simulink model "mod4"  (R2017a)
settings: Solver=VariableStepAuto  StartTime=0.0  StopTime=10.0  RelTol=1e-3
libraries: simulink x2
settings Model: Creator=step_oda  LastModifiedBy=step_oda

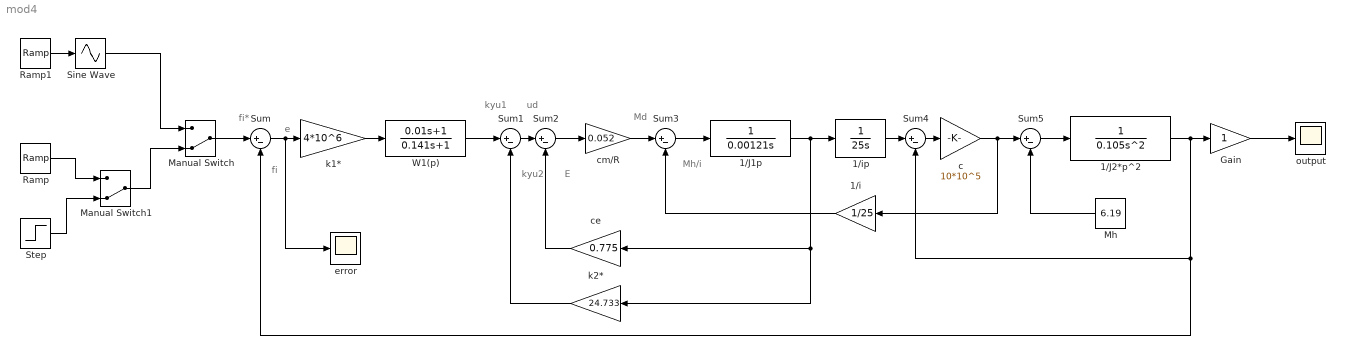
== system mod4 ==
  note: ud
  note: Md
  note: fi
  note: e
  note: fi*
  note: kyu1
  note: kyu2
  note: E
  note: Mh/i
  1/J1p : TransferFcn  Denominator=[0.00121 0]
  1/J2*p^2 : TransferFcn  Denominator=[0.105 0 0]
  1/i : Gain  Gain=1/25
  1/ip : TransferFcn  Denominator=[25 0]
  Gain : Gain
  Manual Switch : ManualSwitch  CurrentSetting=0
  Manual Switch1 : ManualSwitch  CurrentSetting=0
  Mh : Constant  Value=6.19
  Ramp : simulink/Sources/Ramp  slope=4  start=0  X0=0
  Ramp1 : simulink/Sources/Ramp  slope=1  start=0  X0=0
  Sine Wave : Sin  TimeSource=Use external signal  Amplitude=0.533  Frequency=7.5  SampleTime=0
  Step : Step  Time=0  SampleTime=0
  Sum{,1..5} (6 alike) : Sum  Inputs=|+-
  W1(p) : TransferFcn  Numerator=[0.01 1]  Denominator=[0.141 1]
  c : Gain  Gain=10*10^5
  ce : Gain  Gain=0.775
  cm/R : Gain  Gain=0.052
  "error " : Scope
  k1* : Gain  Gain=4*10^6
  k2* : Gain  Gain=24.733
  output : Scope
  wires:
  Manual Switch/1 -> Sum/1
  Sum/1 -> "error "/1, k1*/1
  k1*/1 -> W1(p)/1
  Sum1/1 -> Sum2/1
  Sum3/1 -> 1/J1p/1
  1/J1p/1 -> 1/ip/1, k2*/1, ce/1
  ce/1 -> Sum2/2
  k2*/1 -> Sum1/2
  1/i/1 -> Sum3/2
  Sum2/1 -> cm/R/1
  cm/R/1 -> Sum3/1
  Sine Wave/1 -> Manual Switch/1
  Sum5/1 -> 1/J2*p^2/1
  Sum4/1 -> c/1
  c/1 -> 1/i/1, Sum5/1
  1/ip/1 -> Sum4/1
  1/J2*p^2/1 -> Gain/1, Sum/2, Sum4/2
  Mh/1 -> Sum5/2
  W1(p)/1 -> Sum1/1
  Gain/1 -> output/1
  Ramp1/1 -> Sine Wave/1
  Manual Switch1/1 -> Manual Switch/2
  Ramp/1 -> Manual Switch1/1
  Step/1 -> Manual Switch1/2
